simulink model "TEST_LIDAR"  (R2022b)
settings: Solver=FixedStepAuto  StartTime=0.0  StopTime=inf  FixedStep=1e-3  RelTol=1e-3  EnableMultiTasking=on
model workspace (MAT data in the model file):
  SL_ROS_VariableLengthArrays_MaxSizes : object (value not decoded)
values from neighbouring files (symbols this model uses):
  data = theClient.GetLastFrameOfData()    [FuncMotive.m]
undefined symbols (not defined in the file or in its folder): angular, carstamp, CIRCUIT, CLTF_DAMP, CLTF_FREQ, CLTF_GAIN, CONTROL, CONTROL_INI, DiscIntNeverNeededParam, INPUT, linear, MCP3201, MD25, MODEL, MODEL_INI, mpcstate, MPU60X0, MPU9250, MSG, NAV_MPC_CONTROL, OUTPUT, RCRX, SAMPLING_TIME, SYSID_INPUT, VL6180X
libraries: raspberrypiCommlib x160, simulink x89, raspberrypiNetworklib x22, ros2lib x14, dspsigattribs x14, embedlinuxBasiclib x12, ctrlSharedLib x2, mpclib x1, vrlib x1, sldrtlib x1
(part 14 of 19)

== matlab function TEST_LIDAR/HARDWARE/SENSORS/RCRX iBUS/BUS UPDATE ==
  data: CONTROL_IN input; CONTROL output Bus: CONTROL_Bus; CH_RAW input size=14
function CONTROL = RCRX_UPDATE(CONTROL_IN,CH_RAW)
%--------------------------------------------------------------
% COPY CONTROL BUS
CONTROL = CONTROL_IN;
%--------------------------------------------------------------
% SCALING PARAMETERS
% Open-loop RC scale {'COM MOTOR VOLT','DIFF MOTOR VOLT'}
OPL_RC_SCALE = CONTROL.PARAM.OPL_RC_SCALE;
% Velocity RC scale {'FORWARD VEL REF','YAW RATE REF'}
VEL_RC_SCALE = CONTROL.PARAM.VEL_RC_SCALE;
% Wall follower RC scale {'FORWARD VEL REF','WALL DIST REF'}
WFL_RC_SCALE = CONTROL.PARAM.WFL_RC_SCALE;
% Navigation RC scale {'INC POS X REF','INC POS Y REF'}
NAV_RC_SCALE = CONTROL.PARAM.NAV_RC_SCALE;
%--------------------------------------------------------------
% CHANNEL CALIBRATION
CALIB_PARAM = CONTROL.PARAM.RC_CALIB_PARAM;
CH_TRIM = CONTROL.PARAM.RC_CH_TRIM;
NUM_CH = length(CH_RAW);
CH_PU = zeros(NUM_CH,1);
CH_RAW = double(CH_RAW);
for nn = 1:NUM_CH
    CH_PU(nn) = (CALIB_PARAM(nn,1)*CH_RAW(nn) + CALIB_PARAM(nn,2)).*double(CH_RAW(nn)<CH_TRIM(nn)) + ...
                (CALIB_PARAM(nn,3)*CH_RAW(nn) + CALIB_PARAM(nn,4)).*double(CH_RAW(nn)>=CH_TRIM(nn));
end        
% Channel definition : {'COM MOTOR VOLT','DIFF MOTOR VOLT'}
%                      {'FORWARD VEL REF','YAW RATE REF'}
%                      {'FORWARD VEL REF','YAW ANGLE REF'}
%                      {'FORWARD VEL REF','WALL DIST REF'}
%                      {'INC POS X REF','INC POS Y REF'}
CH_DEF = CONTROL.PARAM.RC_CH_DEF;
% Throttle channel between 0 and 1 
% CH_PU(CH_DEF(4)) = (CH_PU(CH_DEF(4))+1)/2; 
%--------------------------------------------------------------
% TARGET DEFINITION
switch CONTROL.STATE.CONTROL_MODE 
    case 0 % OPEN LOOP
        % {'COMMON MOTOR VOLT','DIFFERENTIAL MOTOR VOLT'}
        if CONTROL.STATE.MV_TARGET_SOURCE(1)==2 % JOYSTICK
            CONTROL.TARGET.MOTOR_VOLT_CD_REF_RC(1) = CH_PU(CH_DEF(1))*OPL_RC_SCALE(1);
        end
        if CONTROL.STATE.MV_TARGET_SOURCE(2)==2 % JOYSTICK
            CONTROL.TARGET.MOTOR_VOLT_CD_REF_RC(2) = CH_PU(CH_DEF(2))*OPL_RC_SCALE(2);
        end
        if CONTROL.STATE.MV_TARGET_SOURCE(1)==3 % SWITCH
            CONTROL.TARGET.MOTOR_VOLT_CD_REF_RC(1) = CONTROL.PARAM.OPL_RC_SWITCH(1,round(2+CH_PU(5)));
        end
        if CONTROL.STATE.MV_TARGET_SOURCE(2)==3 % SWITCH
            CONTROL.TARGET.MOTOR_VOLT_CD_REF_RC(2) = CONTROL.PARAM.OPL_RC_SWITCH(2,round(2+CH_PU(6)));
        end       
    case 1 % FORWARD VELOCITY AND YAW ANGLE
        % {'FORWARD VEL REF','YAW ANGLE REF'}
        if CONTROL.STATE.FV_TARGET_SOURCE==2 % JOYSTICK
            CONTROL.TARGET.FORWARD_VEL_REF_RC = CH_PU(CH_DEF(1))*VEL_RC_SCALE(1);
        end
        if CONTROL.STATE.YA_TARGET_SOURCE==2 % JOYSTICK
            CONTROL.TARGET.YAW_ANG_REF_RC = CH_PU(CH_DEF(2))*VEL_RC_SCALE(2);
        end
        if CONTROL.STATE.FV_TARGET_SOURCE==3 % SWITCH
            CONTROL.TARGET.FORWARD_VEL_REF_RC = CONTROL.PARAM.VEL_RC_SWITCH(1,round(2+CH_PU(5)));
        end
        if CONTROL.STATE.YA_TARGET_SOURCE==3 % SWITCH
            CONTROL.TARGET.YAW_ANG_REF_RC = CONTROL.PARAM.VEL_RC_SWITCH(2,round(2+CH_PU(6)));
        end
    case 2 % FORWARD VELOCITY AND YAW RATE
        % {'FORWARD VEL REF','YAW RATE REF'}
        if CONTROL.STATE.FV_TARGET_SOURCE==2 % JOYSTICK
            CONTROL.TARGET.FORWARD_VEL_REF_RC = CH_PU(CH_DEF(1))*VEL_RC_SCALE(1);
        end
        if CONTROL.STATE.YR_TARGET_SOURCE==2 % JOYSTICK
            CONTROL.TARGET.YAW_RATE_REF_RC = CH_PU(CH_DEF(2))*VEL_RC_SCALE(2);
        end
        if CONTROL.STATE.FV_TARGET_SOURCE==3 % SWITCH
            CONTROL.TARGET.FORWARD_VEL_REF_RC = CONTROL.PARAM.VEL_RC_SWITCH(1,round(2+CH_PU(5)));
        end
        if CONTROL.STATE.YR_TARGET_SOURCE==3 % SWITCH
            CONTROL.TARGET.YAW_RATE_REF_RC = CONTROL.PARAM.VEL_RC_SWITCH(2,round(2+CH_PU(6)));
        end
    case 3 % NAVIGATION
        % {'INC POS X REF','INC POS Y REF'}
        if CONTROL.STATE.NAV_TARGET_SOURCE==2 % JOYSTICK
            CONTROL.TARGET.NAV_REF_RC(1) = CONTROL.INPUT.NAV_MO(1) + CH_PU(CH_DEF(1))*NAV_RC_SCALE;
            CONTROL.TARGET.NAV_REF_RC(2) = CONTROL.INPUT.NAV_MO(2) + CH_PU(CH_DEF(1))*NAV_RC_SCALE;
        end
        if CONTROL.STATE.NAV_TARGET_SOURCE==3 % SWITCH
            % CONTROL.TARGET.NAV_REF_RC(1) = CONTROL.INPUT.NAV_MO(1) + CONTROL.PARAM.NAV_RC_SWITCH(1,round(2+CH_PU(5)));
            % CONTROL.TARGET.NAV_REF_RC(2) = CONTROL.INPUT.NAV_MO(2) + CONTROL.PARAM.NAV_RC_SWITCH(2,round(2+CH_PU(6)));
            CONTROL.TARGET.NAV_REF_RC(1) = CONTROL.PARAM.NAV_RC_SWITCH(1,round(2+CH_PU(5)));
            CONTROL.TARGET.NAV_REF_RC(2) = CONTROL.PARAM.NAV_RC_SWITCH(2,round(2+CH_PU(6)));
        end
    case {4,5} % WALL FOLLOWER
        % {'FORWARD VEL REF','WALL DIST REF'}
        if CONTROL.STATE.FV_TARGET_SOURCE==2 % JOYSTICK
            CONTROL.TARGET.FORWARD_VEL_REF_RC = CH_PU(CH_DEF(1))*WFL_RC_SCALE(1);
        end
        % {'FORWARD VEL REF','WALL DIST REF'}
        if CONTROL.STATE.WD_TARGET_SOURCE==2 % JOYSTICK
            CONTROL.TARGET.WALL_DIST_REF_RC = 0.1 + CH_PU(CH_DEF(2))*WFL_RC_SCALE(2);
        end
        if CONTROL.STATE.FV_TARGET_SOURCE==3 % SWITCH
            CONTROL.TARGET.FORWARD_VEL_REF_RC = CONTROL.PARAM.WFL_RC_SWITCH(1,round(2+CH_PU(5)));
        end
        if CONTROL.STATE.WD_TARGET_SOURCE==3 % SWITCH
            CONTROL.TARGET.WALL_DIST_REF_RC = CONTROL.PARAM.WFL_RC_SWITCH(2,round(2+CH_PU(6)));
        end
    otherwise % FORWARD VELOCITY AND YAW RATE
        % {'FORWARD VEL REF','YAW RATE REF'}
        if CONTROL.STATE.FV_TARGET_SOURCE==2 % JOYSTICK
            CONTROL.TARGET.FORWARD_VEL_REF_RC = CH_PU(CH_DEF(1))*VEL_RC_SCALE(1);
        end
        if CONTROL.STATE.YR_TARGET_SOURCE==2 % JOYSTICK
            CONTROL.TARGET.YAW_RATE_REF_RC = CH_PU(CH_DEF(2))*VEL_RC_SCALE(1);
        end
        if CONTROL.STATE.FV_TARGET_SOURCE==3 % SWITCH
            CONTROL.TARGET.FORWARD_VEL_REF_RC = CONTROL.PARAM.VEL_RC_SWITCH(1,round(2+CH_PU(5)));
        end
        if CONTROL.STATE.YR_TARGET_SOURCE==3 % SWITCH
            CONTROL.TARGET.YAW_RATE_REF_RC = CONTROL.PARAM.VEL_RC_SWITCH(2,round(2+CH_PU(6)));
        end
end
if abs(CONTROL.TARGET.MOTOR_VOLT_CD_REF_RC(1))<0.25
    CONTROL.TARGET.MOTOR_VOLT_CD_REF_RC(1) = 0;
end
if abs(CONTROL.TARGET.MOTOR_VOLT_CD_REF_RC(2))<0.25
    CONTROL.TARGET.MOTOR_VOLT_CD_REF_RC(2) = 0;
end
if abs(CONTROL.TARGET.FORWARD_VEL_REF_RC)<0.05
    CONTROL.TARGET.FORWARD_VEL_REF_RC = 0;
end
if abs(CONTROL.TARGET.YAW_RATE_REF_RC)<0.025
    CONTROL.TARGET.YAW_RATE_REF_RC = 0;
end
%--------------------------------------------------------------
% CONTROL BUS UPDATE
% RC CHANNELS (pu): channel range [-1 1] / Throtle range (channel 4) [0 1] 
CONTROL.TARGET.RC_CH_PU = CH_PU(:);
CONTROL.TARGET.RC_CH_RAW = CH_RAW(:);

== matlab function TEST_LIDAR/HARDWARE/SENSORS/RCRX iBUS/MATLAB Function ==
  data: iBUS_DATA input; CH_RAW output size=14
function CH_RAW = iBUS_DECODER(iBUS_DATA)
%--------------------------------------------------------------
persistent initialize CH_RAW_PREV
if isempty(initialize)
    initialize = 1;
    CH_RAW_PREV = uint16(1500*ones(14,1));
end
%--------------------------------------------------------------
% iBUS protocol: 14 channels uint16 in the range [1000 - 2000]
%--------------------------------------------------------------
% HEADER DETECTION
header = uint8([32 64]);
AUX1 = (iBUS_DATA == header(1));
AUX2 = (iBUS_DATA == header(2));
AUX3 = AUX1(1:end-1) & AUX2(2:end);
[max_value,index] = max(AUX3);
%--------------------------------------------------------------
% CHANNEL DETECTION
if max_value && ((index(1)+2+2*14-1)<=length(iBUS_DATA))
    CH_DATA = iBUS_DATA((index(1)+2):(index(1)+2+2*14-1));
    CH_LSB = uint16(CH_DATA(1:2:length(CH_DATA)));
    CH_MSB = uint16(CH_DATA(2:2:length(CH_DATA)));
    CH_RAW_AUX = uint16(CH_MSB*2^8 + CH_LSB);
    CH_RAW_PREV = CH_RAW_AUX;
else
    CH_RAW_AUX = CH_RAW_PREV;
end

CH_RAW = CH_RAW_AUX(1:14);

return

== matlab function TEST_LIDAR/GAZEBO SIMULATION/COMMUNICATIONS/BT_RX/MCS RX ==
  data: CONTROL_IN input; BUFFER_RX_LAST input; CONTROL output Bus: CONTROL_Bus; STATUS input
function CONTROL  = MCS_DECODER(CONTROL_IN,BUFFER_RX_LAST,STATUS)
                 
persistent BUFFER_RX PAYLOAD
if isempty(BUFFER_RX)
    BUFFER_RX = zeros(50,3,'uint8');
    PAYLOAD = zeros(26,1,'uint8');
end

% Initialization
MESSAGE_LEN = length(PAYLOAD);
CONTROL = CONTROL_IN;
[BUFFER_ROW,BUFFER_COL] = size(BUFFER_RX);
% Update buffer
BUFFER_RX_VEC = [BUFFER_RX(:) ; BUFFER_RX_LAST];
BUFFER_LEN = length(BUFFER_RX_VEC);
% Identify sequences [13 10 254]
IDX_AUX = find(BUFFER_RX_VEC(1:end-2)==uint8(13) & BUFFER_RX_VEC(2:end-1)==uint8(10) & BUFFER_RX_VEC(3:end)==uint8(254));
if isempty(IDX_AUX) 
    % There is not any message
    flag_msg = false;
    BUFFER_RX = zeros(size(BUFFER_RX),'uint8');
    return
elseif IDX_AUX(1)+MESSAGE_LEN+2>BUFFER_LEN 
    % There is 1 incomplete message 
    flag_msg = false;
    BUFFER_RX = [BUFFER_RX(:,2:end)  BUFFER_RX_LAST];
    return
else
    % There is 1 complete message at least  
    flag_msg = true;
    IDX_START = zeros(size(IDX_AUX));
    IDX_END = zeros(size(IDX_AUX));
    IDX_AUX = [IDX_AUX ; BUFFER_LEN];
    IDX_START(1) = IDX_AUX(1) + 3;
    IDX_END(1) = IDX_START(1) + MESSAGE_LEN - 1;    
    COUNT = 1;
    % The rest of sequences [13 10 254] are verified
    for nn = 2:length(IDX_AUX)-1
        if (IDX_END(COUNT) < IDX_AUX(nn)) && (IDX_AUX(nn)+3<BUFFER_LEN)
            if IDX_AUX(nn) + MESSAGE_LEN + 1 <= BUFFER_LEN
                COUNT = COUNT +1;
                IDX_START(COUNT) = IDX_AUX(nn) + 3;
                IDX_END(COUNT) = IDX_START(COUNT) + MESSAGE_LEN - 1;       
            end
        end
    end
end
IDX_START = IDX_START(1:COUNT);
IDX_END = IDX_END(1:COUNT);
% Message identification
NUM_MESSAGES = COUNT;
MESSAGE = cell(NUM_MESSAGES,1);
for COUNT = 1:NUM_MESSAGES
    % Message building
    MESSAGE{COUNT} = BUFFER_RX_VEC(IDX_START(COUNT):IDX_END(COUNT));
end
% Update BUFFER_RX
BUFFER_RX_VEC = [zeros(IDX_END(end)-BUFFER_ROW-1,1,'uint8') ; BUFFER_RX_VEC(IDX_END(end):end)];
for nn = 1:BUFFER_COL
    BUFFER_RX(:,nn) = BUFFER_RX_VEC((nn-1)*BUFFER_ROW+1:BUFFER_ROW*nn);
end

%%%%%%%%%%%%%%%%%%%%%%%%%%%%%%%%%%%%%%%%%%%%%%%%%%%%%%%%%%%%%%%%%%%%%%%%%%%
% MCS MESSAGES
%%%%%%%%%%%%%%%%%%%%%%%%%%%%%%%%%%%%%%%%%%%%%%%%%%%%%%%%%%%%%%%%%%%%%%%%%%%
if flag_msg && STATUS==0
    PAYLOAD(1:MESSAGE_LEN) = uint8(MESSAGE{end});
end
% CRC    
CRC_VALUE=uint16(65535);
for nn=1:MESSAGE_LEN-2
    TMP=bitxor(uint16(PAYLOAD(nn)),bitand(CRC_VALUE,uint16(255)));
    TMP4=bitand(bitshift(TMP,4),uint16(255));
    TMP=bitxor(TMP,TMP4);
    TMP8=bitshift(TMP,8);
    TMP3=bitshift(TMP,3);
    TMP_4=bitshift(TMP,-4);
    CRC_VALUE=bitxor(bitshift(CRC_VALUE,-8),bitxor(TMP8,bitxor(TMP3,TMP_4)));
    CRC_VALUE=bitand(CRC_VALUE,uint16(65535));
end
CRC1=uint8(bitand(CRC_VALUE,uint16(255)));
CRC2=uint8(bitand(bitshift(CRC_VALUE,-8),uint16(255)));

% CRC checking
if (CRC1 == PAYLOAD(MESSAGE_LEN-1))  && (CRC2 == PAYLOAD(MESSAGE_LEN))
    % WRITE IN THE CONTROL BUS
    CONTROL.INPUT.MCS_EARTH_POS(1) = double(typecast(PAYLOAD(1:4),'single'));
    CONTROL.INPUT.MCS_EARTH_POS(2) = double(typecast(PAYLOAD(5:8),'single'));
    CONTROL.INPUT.MCS_EARTH_POS(3) = double(typecast(PAYLOAD(9:12),'single'));
    CONTROL.INPUT.MCS_EULER_ANG(1) = double(typecast(PAYLOAD(13:16),'single'));
    CONTROL.INPUT.MCS_EULER_ANG(2) = double(typecast(PAYLOAD(17:20),'single'));
    CONTROL.INPUT.MCS_EULER_ANG(3) = double(typecast(PAYLOAD(21:24),'single'));

    % UNWRAPPING
    aux1 = CONTROL.INPUT.MCS_EULER_ANG(3);
    aux2 = CONTROL.TARGET.YAW_ANG_REF;
    INC_ANG = zeros(41,1);
    INC_ANG(1) = aux1-aux2;
    for ii = 1:20
        INC_ANG(2*ii)   = aux1-aux2-2*ii*pi;
        INC_ANG(2*ii+1) = aux1-aux2+2*ii*pi;
    end
    [~,ind] = min(abs(INC_ANG));
    NAV_YAW_ANG = aux2 + INC_ANG(ind);
    CONTROL.INPUT.MCS_EULER_ANG(3) = NAV_YAW_ANG;

    % POSITION CORRECTION
    % rv = rm + rc*exp(Shi*j)
    % xv = xm + xc*cos(Shi);
    % yv = ym + yc*sin(Shi);
    CONTROL.INPUT.MCS_EARTH_POS(1) = CONTROL.INPUT.MCS_EARTH_POS(1) - CONTROL.PARAM.NAV_CENTER_POS(1)*cos(CONTROL.INPUT.MCS_EULER_ANG(3));
    CONTROL.INPUT.MCS_EARTH_POS(2) = CONTROL.INPUT.MCS_EARTH_POS(2) - CONTROL.PARAM.NAV_CENTER_POS(2)*sin(CONTROL.INPUT.MCS_EULER_ANG(3));

    % INITIAL POSITION COMPENSATION
    if CONTROL.STATE.CURRENT_STATUS_SYS>1
        CONTROL.INPUT.MCS_EARTH_POS = CONTROL.INPUT.MCS_EARTH_POS - CONTROL.PARAM.MCS_EARTH_POS_OFFS;
        CONTROL.INPUT.MCS_EULER_ANG = CONTROL.INPUT.MCS_EULER_ANG - CONTROL.PARAM.MCS_EULER_ANG_OFFS;
    end
    
end
%%%%%%%%%%%%%%%%%%%%%%%%%%%%%%%%%%%%%%%%%%%%%%%%%%%%%%%%%%%%%%%%%%%%%%%%%%%


return

== matlab function TEST_LIDAR/CONTROL/LOCAL TARGETS/FORWARD VELOCITY TARGET/ PULSE GENERATION ==
  data: CONTROL input Bus: CONTROL_Bus; FORWARD_VEL_REF output
function FORWARD_VEL_REF = PULSE_GEN(CONTROL)
    
persistent TIMER initialize
if isempty(initialize)
    TIMER = 0;
    initialize = 1;
end

% SAMPLING TIME
SAMPLING_TIME = CONTROL.PARAM.SAMPLING_TIME; % s

%% OPERATION MODE
% / 0. BOOTING   / 1. SENSOR CALIBRATION / 2. READY
% / 3. OPEN LOOP / 4. ATTITUDE / 5. VELOCITY / 6. NAVIGATION / 
% / 7. WALL FOLLOWER / 8. WALL-FOLLOWER COMPETITION / 
% / 9. NAVIGATION COMPETITION / 10. STOP
CURRENT_STATUS = CONTROL.STATE.CURRENT_STATUS_SYS;
PREVIOUS_STATUS = CONTROL.STATE.PREVIOUS_STATUS;

if (CURRENT_STATUS == 5) && (PREVIOUS_STATUS == 5)   
    if TIMER > 7.5
        FORWARD_VEL_REF = 0;
    elseif TIMER < 5
        FORWARD_VEL_REF = 0;
        TIMER = TIMER + SAMPLING_TIME;
    else % 5 <= TIMER <= 7.5
        FORWARD_VEL_REF = 0.25;
        TIMER = TIMER + SAMPLING_TIME;
    end
else
    FORWARD_VEL_REF = 0;
    TIMER = 0;
end

== matlab function TEST_LIDAR/CONTROL/LOCAL TARGETS/YAW RATE TARGET/ PULSE GENERATION  ==
  data: CONTROL input Bus: CONTROL_Bus; YAW_RATE_REF output
function YAW_RATE_REF = PULSE_GEN(CONTROL)
    
persistent TIMER initialize
if isempty(initialize)
    TIMER = 0;
    initialize = 1;
end

% SAMPLING TIME
SAMPLING_TIME = CONTROL.PARAM.SAMPLING_TIME; % s

%% OPERATION MODE
% / 0. BOOTING   / 1. SENSOR CALIBRATION / 2. READY
% / 3. OPEN LOOP / 4. ATTITUDE / 5. VELOCITY / 6. NAVIGATION / 
% / 7. WALL FOLLOWER / 8. WALL-FOLLOWER COMPETITION / 
% / 9. NAVIGATION COMPETITION / 10. STOP
CURRENT_STATUS = CONTROL.STATE.CURRENT_STATUS_SYS;
PREVIOUS_STATUS = CONTROL.STATE.PREVIOUS_STATUS;

if (CURRENT_STATUS == 5) && (PREVIOUS_STATUS == 5)   
    if TIMER > 7.5
        YAW_RATE_REF = 0;
    elseif TIMER < 5
        YAW_RATE_REF = 0;
        TIMER = TIMER + SAMPLING_TIME;
    else % 5 <= TIMER <= 7.5
        YAW_RATE_REF = 30*pi/180;
        TIMER = TIMER + SAMPLING_TIME;
    end
else
    YAW_RATE_REF = 0;
    TIMER = 0;
end

== matlab function TEST_LIDAR/SIMULATION/CIRCUIT SIMULATION ==
  data: MODEL_IN input; MODEL output Bus: MODEL_Bus
function MODEL = CIRCUIT_SIM(MODEL_IN)
% function [d,theta_circ,d1,d2,rampa,estado] = CIRCUIT_SIM(xi,yi,theta,param,est_ant)

% PARAMETERS
MODEL.CIRCUIT.PERIMETER_POINTS = 1000;
MODEL.CIRCUIT.STRAIGHT_SIDE_LENGTH = 2;
MODEL.CIRCUIT.RAMP_LENGTH = 1.5;
MODEL.CIRCUIT.CURVE_RADIUS = 0.5;
MODEL.CIRCUIT.RAMP = 0;
MODEL.CIRCUIT.STATUS = 0;

L=param(1); % Longitud tramo recto
Lr=param(2); % Longitud rampa
R=param(3);  % Radio de la curva
d_sens=param(4); % Distancia entre sensores

% Sensor delantero
xid=xi+d_sens/2*cos(theta);
yid=yi+d_sens/2*sin(theta);
% Sensor trasero
xit=xi-d_sens/2*cos(theta);
yit=yi-d_sens/2*sin(theta);
% Ecuacion de la recta normal
% y-yi = tan(theta-pi/2)*(x-xi)

%% Distancia del sensor delantero
% Corte con el tramo recto de la pared del circuito
% x=xi+(sign(yi)*R-yi)/tan(theta-pi/2)
x_1=[xid+(R-yid)/tan(theta-pi/2); xid+(-R-yid)/tan(theta-pi/2)];
y_1=[R; -R];
V1=(x_1-xid)+1j*(y_1-yid);
V2=d_sens/2*cos(theta)+1j*d_sens/2*sin(theta);
ang_1=angle(V2./V1)*180/pi;
[~,ind]=min(abs(ang_1-90));
x_1=x_1(ind);
y_1=y_1(ind);
% Corte con la curva del circuito
% (yi+tan(theta-pi/2)*(x-xi))^2 = R^2-(x-sign(xi)*L/2)^2
% yi^2+tan(theta-pi/2)^2*(x^2+xi^2-2*xi*x)+2*tan(theta-pi/2)*(x-xi)*yi = R^2-x^2-L^2/4+2*sign(xi)*L/2*x
% x = roots([tan(theta-pi/2)^2+1  -2*(xi*tan(theta-pi/2)^2+sign(xi)*L/2-tan(theta-pi/2)*yi)   yi^2+tan(theta-pi/2)^2*xi^2-R^2+L^2/4-2*tan(theta-pi/2)*xi*yi])
if abs(x_1)<=L/2
    xcd=x_1;
    ycd=y_1;
else
    x_2 = roots([tan(theta-pi/2)^2+1 ...
        -2*(xid*tan(theta-pi/2)^2+sign(xid)*L/2-tan(theta-pi/2)*yid) ...
        yid^2+tan(theta-pi/2)^2*xid^2-R^2+L^2/4-2*tan(theta-pi/2)*xid*yid]);
        [~,ind]=min(abs(x_2-xid));
    xcd=x_2(ind);
    aux=sqrt(abs(R^2-(xcd-sign(xid)*L/2)^2));
    y_2=[aux ; -aux];
    V1=[(xcd-xid)+1j*(y_2(1)-yid) ; (xcd-xid)+1j*(y_2(2)-yid)];
    V2=[d_sens/2*cos(theta)+1j*d_sens/2*sin(theta); d_sens/2*cos(theta)+1j*d_sens/2*sin(theta)];
    ang_2=angle(V2./V1)*180/pi;
    [~,ind]=min(abs(ang_2-90));
    ycd=y_2(ind);
end
d1=norm([xcd-xid ; ycd-yid]);

%% Distancia del sensor trasero
% Corte con el tramo recto de la pared del circuito
% x=xi+(sign(yi)*R-yi)/tan(theta-pi/2)
x_1=[xit+(R-yit)/tan(theta-pi/2); xit+(-R-yit)/tan(theta-pi/2)];
y_1=[R; -R];
V1=(x_1-xit)+1j*(y_1-yit);
V2=d_sens/2*cos(theta)+1j*d_sens/2*sin(theta);
ang_1=angle(V2./V1)*180/pi;
[~,ind]=min(abs(ang_1-90));
x_1=x_1(ind);
y_1=y_1(ind);
% Corte con la curva del circuito
% (yi+tan(theta-pi/2)*(x-xi))^2 = R^2-(x-sign(xi)*L/2)^2
% yi^2+tan(theta-pi/2)^2*(x^2+xi^2-2*xi*x)+2*tan(theta-pi/2)*(x-xi)*yi = R^2-x^2-L^2/4+2*sign(xi)*L/2*x
% x = roots([tan(theta-pi/2)^2+1  -2*(xi*tan(theta-pi/2)^2+sign(xi)*L/2-tan(theta-pi/2)*yi)   yi^2+tan(theta-pi/2)^2*xi^2-R^2+L^2/4-2*tan(theta-pi/2)*xi*yi])
if abs(x_1)<=L/2
    xct=x_1;
    yct=y_1;
else
    x_2 = roots([tan(theta-pi/2)^2+1 ...
        -2*(xit*tan(theta-pi/2)^2+sign(xit)*L/2-tan(theta-pi/2)*yit) ...
        yit^2+tan(theta-pi/2)^2*xit^2-R^2+L^2/4-2*tan(theta-pi/2)*xit*yit]);
        [~,ind]=min(abs(x_2-xit));
    xct=x_2(ind);
    aux=sqrt(abs(R^2-(xct-sign(xit)*L/2)^2));
    y_2=[aux ; -aux];
    V1=[(xct-xit)+1j*(y_2(1)-yit) ; (xct-xit)+1j*(y_2(2)-yit)];
    V2=[d_sens/2*cos(theta)+1j*d_sens/2*sin(theta); d_sens/2*cos(theta)+1j*d_sens/2*sin(theta)];
    ang_2=angle(V2./V1)*180/pi;
    [~,ind]=min(abs(ang_2-90));
    yct=y_2(ind);
end
d2=norm([xct-xit ; yct-yit]);

%% Angulo con respecto al circuito
theta_circ=atan2(d1-d2,d_sens);

%% Distancia en m
d=(d1+d2)/2/cosd(theta_circ);
d1=d1;
d2=d2;

% Existencia de rampa
rampa=0;
if abs(xi)<=Lr/2 
   % El coche está en la rampa
   if yi<0
       % Rampa ascendente
       rampa=1;
   else
       % Rampa descendente
       rampa=-1;
   end
end
% Determinacion del estado
if abs(xi)<=L/2 
   % El coche está en el tramo recto
   if yi<0
       % Subida
       estado=est_ant+(rem(est_ant,4)==1);
   else
       % Bajada
       estado=est_ant+(rem(est_ant,4)==3);
   end
elseif xi>L/2
    % El coche está en la curva superior
       estado=est_ant+(rem(est_ant,4)==2);
else
    % El coche está en la curva inferior
    estado=est_ant+(rem(est_ant,4)==0);
end

== matlab function TEST_LIDAR/HARDWARE/COMMUNICATIONS/BT_RX/MCS RX ==
  data: CONTROL_IN input; BUFFER_RX_LAST input; CONTROL output Bus: CONTROL_Bus; STATUS input
function CONTROL  = MCS_DECODER(CONTROL_IN,BUFFER_RX_LAST,STATUS)
                 
persistent BUFFER_RX PAYLOAD
if isempty(BUFFER_RX)
    BUFFER_RX = zeros(50,3,'uint8');
    PAYLOAD = zeros(26,1,'uint8');
end

% Initialization
MESSAGE_LEN = length(PAYLOAD);
CONTROL = CONTROL_IN;
[BUFFER_ROW,BUFFER_COL] = size(BUFFER_RX);
% Update buffer
BUFFER_RX_VEC = [BUFFER_RX(:) ; BUFFER_RX_LAST];
BUFFER_LEN = length(BUFFER_RX_VEC);
% Identify sequences [13 10 254]
IDX_AUX = find(BUFFER_RX_VEC(1:end-2)==uint8(13) & BUFFER_RX_VEC(2:end-1)==uint8(10) & BUFFER_RX_VEC(3:end)==uint8(254));
if isempty(IDX_AUX) 
    % There is not any message
    flag_msg = false;
    BUFFER_RX = zeros(size(BUFFER_RX),'uint8');
    return
elseif IDX_AUX(1)+MESSAGE_LEN+2>BUFFER_LEN 
    % There is 1 incomplete message 
    flag_msg = false;
    BUFFER_RX = [BUFFER_RX(:,2:end)  BUFFER_RX_LAST];
    return
else
    % There is 1 complete message at least  
    flag_msg = true;
    IDX_START = zeros(size(IDX_AUX));
    IDX_END = zeros(size(IDX_AUX));
    IDX_AUX = [IDX_AUX ; BUFFER_LEN];
    IDX_START(1) = IDX_AUX(1) + 3;
    IDX_END(1) = IDX_START(1) + MESSAGE_LEN - 1;    
    COUNT = 1;
    % The rest of sequences [13 10 254] are verified
    for nn = 2:length(IDX_AUX)-1
        if (IDX_END(COUNT) < IDX_AUX(nn)) && (IDX_AUX(nn)+3<BUFFER_LEN)
            if IDX_AUX(nn) + MESSAGE_LEN + 1 <= BUFFER_LEN
                COUNT = COUNT +1;
                IDX_START(COUNT) = IDX_AUX(nn) + 3;
                IDX_END(COUNT) = IDX_START(COUNT) + MESSAGE_LEN - 1;       
            end
        end
    end
end
IDX_START = IDX_START(1:COUNT);
IDX_END = IDX_END(1:COUNT);
% Message identification
NUM_MESSAGES = COUNT;
MESSAGE = cell(NUM_MESSAGES,1);
for COUNT = 1:NUM_MESSAGES
    % Message building
    MESSAGE{COUNT} = BUFFER_RX_VEC(IDX_START(COUNT):IDX_END(COUNT));
end
% Update BUFFER_RX
BUFFER_RX_VEC = [zeros(IDX_END(end)-BUFFER_ROW-1,1,'uint8') ; BUFFER_RX_VEC(IDX_END(end):end)];
for nn = 1:BUFFER_COL
    BUFFER_RX(:,nn) = BUFFER_RX_VEC((nn-1)*BUFFER_ROW+1:BUFFER_ROW*nn);
end

%%%%%%%%%%%%%%%%%%%%%%%%%%%%%%%%%%%%%%%%%%%%%%%%%%%%%%%%%%%%%%%%%%%%%%%%%%%
% MCS MESSAGES
%%%%%%%%%%%%%%%%%%%%%%%%%%%%%%%%%%%%%%%%%%%%%%%%%%%%%%%%%%%%%%%%%%%%%%%%%%%
if flag_msg && STATUS==0
    PAYLOAD(1:MESSAGE_LEN) = uint8(MESSAGE{end});
end
% CRC    
CRC_VALUE=uint16(65535);
for nn=1:MESSAGE_LEN-2
    TMP=bitxor(uint16(PAYLOAD(nn)),bitand(CRC_VALUE,uint16(255)));
    TMP4=bitand(bitshift(TMP,4),uint16(255));
    TMP=bitxor(TMP,TMP4);
    TMP8=bitshift(TMP,8);
    TMP3=bitshift(TMP,3);
    TMP_4=bitshift(TMP,-4);
    CRC_VALUE=bitxor(bitshift(CRC_VALUE,-8),bitxor(TMP8,bitxor(TMP3,TMP_4)));
    CRC_VALUE=bitand(CRC_VALUE,uint16(65535));
end
CRC1=uint8(bitand(CRC_VALUE,uint16(255)));
CRC2=uint8(bitand(bitshift(CRC_VALUE,-8),uint16(255)));

% CRC checking
if (CRC1 == PAYLOAD(MESSAGE_LEN-1))  && (CRC2 == PAYLOAD(MESSAGE_LEN))
    % WRITE IN THE CONTROL BUS
    CONTROL.INPUT.MCS_EARTH_POS(1) = double(typecast(PAYLOAD(1:4),'single'));
    CONTROL.INPUT.MCS_EARTH_POS(2) = double(typecast(PAYLOAD(5:8),'single'));
    CONTROL.INPUT.MCS_EARTH_POS(3) = double(typecast(PAYLOAD(9:12),'single'));
    CONTROL.INPUT.MCS_EULER_ANG(1) = double(typecast(PAYLOAD(13:16),'single'));
    CONTROL.INPUT.MCS_EULER_ANG(2) = double(typecast(PAYLOAD(17:20),'single'));
    CONTROL.INPUT.MCS_EULER_ANG(3) = double(typecast(PAYLOAD(21:24),'single'));

    % UNWRAPPING
    aux1 = CONTROL.INPUT.MCS_EULER_ANG(3);
    aux2 = CONTROL.TARGET.YAW_ANG_REF;
    INC_ANG = zeros(41,1);
    INC_ANG(1) = aux1-aux2;
    for ii = 1:20
        INC_ANG(2*ii)   = aux1-aux2-2*ii*pi;
        INC_ANG(2*ii+1) = aux1-aux2+2*ii*pi;
    end
    [~,ind] = min(abs(INC_ANG));
    NAV_YAW_ANG = aux2 + INC_ANG(ind);
    CONTROL.INPUT.MCS_EULER_ANG(3) = NAV_YAW_ANG;

    % POSITION CORRECTION
    % rv = rm + rc*exp(Shi*j)
    % xv = xm + xc*cos(Shi);
    % yv = ym + yc*sin(Shi);
    CONTROL.INPUT.MCS_EARTH_POS(1) = CONTROL.INPUT.MCS_EARTH_POS(1) - CONTROL.PARAM.NAV_CENTER_POS(1)*cos(CONTROL.INPUT.MCS_EULER_ANG(3));
    CONTROL.INPUT.MCS_EARTH_POS(2) = CONTROL.INPUT.MCS_EARTH_POS(2) - CONTROL.PARAM.NAV_CENTER_POS(2)*sin(CONTROL.INPUT.MCS_EULER_ANG(3));

    % INITIAL POSITION COMPENSATION
    if CONTROL.STATE.CURRENT_STATUS_SYS>1
        CONTROL.INPUT.MCS_EARTH_POS = CONTROL.INPUT.MCS_EARTH_POS - CONTROL.PARAM.MCS_EARTH_POS_OFFS;
        CONTROL.INPUT.MCS_EULER_ANG = CONTROL.INPUT.MCS_EULER_ANG - CONTROL.PARAM.MCS_EULER_ANG_OFFS;
    end
    
end
%%%%%%%%%%%%%%%%%%%%%%%%%%%%%%%%%%%%%%%%%%%%%%%%%%%%%%%%%%%%%%%%%%%%%%%%%%%


return

== matlab function TEST_LIDAR/HARDWARE/ACTUATORS/MD25_I2C/READ BATTERY VOLTAGE/BATTERY VOLTAGE FILTER ==
  data: CONTROL_IN input; BATTERY_VOLT input; CONTROL output Bus: CONTROL_Bus; RATED_BATTERY_VOLT input; THR_NLFILT input; ALFA_FILT input
function CONTROL = BATTERY_VOLT_FILTER(CONTROL_IN,BATTERY_VOLT,RATED_BATTERY_VOLT,THR_NLFILT,ALFA_FILT)

%--------------------------------------------------------------
% COPY CONTROL BUS
%--------------------------------------------------------------
CONTROL = CONTROL_IN;

%--------------------------------------------------------------
% STATE
%--------------------------------------------------------------
persistent initialize BATTERY_VOLT_NLFILT BATTERY_VOLT_FILT
if isempty(initialize)
    BATTERY_VOLT_NLFILT = RATED_BATTERY_VOLT;
    BATTERY_VOLT_FILT = RATED_BATTERY_VOLT;
    initialize = 1;
end

%--------------------------------------------------------------
% NON-LINEAR FILTER
%--------------------------------------------------------------
if abs(BATTERY_VOLT - BATTERY_VOLT_NLFILT) < THR_NLFILT
    BATTERY_VOLT_NLFILT = BATTERY_VOLT;
end

%--------------------------------------------------------------
% FIRST-ORDER LINEAR FILTER
%--------------------------------------------------------------
BATTERY_VOLT_FILT = ALFA_FILT*BATTERY_VOLT_FILT + (1-ALFA_FILT)*BATTERY_VOLT_NLFILT;

%--------------------------------------------------------------
% CONTROL BUS UPDATE
%--------------------------------------------------------------
CONTROL.INPUT.BATTERY_VOLT = BATTERY_VOLT_FILT; % V   

return

== matlab function TEST_LIDAR/HARDWARE/ACTUATORS/MD25_I2C/READ MOTOR ENCODER/READ ENCODER ANGLE ==
  data: CONTROL_IN input; MOTOR_ENC_BYTES input uint8; CONTROL output CONTROL_Bus
function CONTROL = READ_ENCODER_ANGLE(CONTROL_IN,MOTOR_ENC_BYTES)

%--------------------------------------------------------------
% COPY CONTROL BUS
%--------------------------------------------------------------
CONTROL = CONTROL_IN;

%--------------------------------------------------------------
% PARAMETERS
%--------------------------------------------------------------
% Sampling time (s)
SAMPLING_TIME = CONTROL.PARAM.SAMPLING_TIME;
% Encoder filter frequency (Hz)
ENC_FILT_FREQ = CONTROL.PARAM.ENC_FILT_FREQ;
% Distance between wheeels (m)
WHEEL_DIST = CONTROL.PARAM.WHEEL_DISTANCE;
% Wheel radius (m)
WHEEL_RADIUS = CONTROL.PARAM.WHEEL_RADIUS;
% Wheel gear ratio
WHEEL_GEAR_RATIO = CONTROL.PARAM.WHEEL_GEAR_RATIO;
% Motor gear ratio
MOTOR_GEAR_RATIO = CONTROL.PARAM.MOTOR_GEAR_RATIO;
% Encoder resolution: number of pulses / revolution of main shaft
MOTOR_ENC_RES = CONTROL.PARAM.MOTOR_ENC_RES; 

%--------------------------------------------------------------
% ENCODER READOUT
%--------------------------------------------------------------
MOTOR_ENC_COUNT = zeros(2,1);
MOTOR_ENC_COUNT(1) = -double(typecast(MOTOR_ENC_BYTES([4 3 2 1],1),'int32'));
MOTOR_ENC_COUNT(2) = -double(typecast(MOTOR_ENC_BYTES([8 7 6 5],1),'int32'));

%--------------------------------------------------------------
% STATE
%--------------------------------------------------------------
persistent initialize INC_ENC_FILT ENC_COUNT_NLFILT YAW_ANGLE YAW_ANGLE_FILT...
           YAW_RATE YAW_RATE_FILT
if isempty(initialize)
    YAW_ANGLE = 0;
    YAW_RATE = 0;
    YAW_ANGLE_FILT = 0;
    YAW_RATE_FILT = 0;
    INC_ENC_FILT = zeros(2,1); 
    ENC_COUNT_NLFILT = MOTOR_ENC_COUNT;
    initialize = 1;
end

%--------------------------------------------------------------
% NON-LINEAR FILTER
%--------------------------------------------------------------
LAST_ENC_COUNT_NLFILT = ENC_COUNT_NLFILT;
MOTOR_ENC_COUNT_INC = MOTOR_ENC_COUNT - ENC_COUNT_NLFILT;
AUX = abs(MOTOR_ENC_COUNT)>0 & abs(MOTOR_ENC_COUNT_INC)<50;
if AUX(1)
    ENC_COUNT_NLFILT(1) = MOTOR_ENC_COUNT(1);
end
if AUX(2)
    ENC_COUNT_NLFILT(2) = MOTOR_ENC_COUNT(2);
end

%--------------------------------------------------------------
% LINEAR FILTER APPLIED TO INCREMENTAL ENCODER COUNT
%--------------------------------------------------------------
INC_ENC = ENC_COUNT_NLFILT - LAST_ENC_COUNT_NLFILT;
% LPF discrete-time pole
ALFA = exp(-SAMPLING_TIME*2*pi*ENC_FILT_FREQ);
INC_ENC_FILT = ALFA*INC_ENC_FILT + (1-ALFA)*INC_ENC;  

%--------------------------------------------------------------
% FORWARD VELOCITY
%--------------------------------------------------------------
FORWARD_VEL = mean(INC_ENC)/MOTOR_ENC_RES*2*pi/SAMPLING_TIME/MOTOR_GEAR_RATIO/WHEEL_GEAR_RATIO*WHEEL_RADIUS;
FORWARD_VEL_FILT = mean(INC_ENC_FILT)/MOTOR_ENC_RES*2*pi/SAMPLING_TIME/MOTOR_GEAR_RATIO/WHEEL_GEAR_RATIO*WHEEL_RADIUS;

%--------------------------------------------------------------
% YAW RATE
%--------------------------------------------------------------
YAW_RATE_PRV = YAW_RATE;
YAW_RATE_PRV_FILT = YAW_RATE_FILT;
YAW_RATE = (INC_ENC(1)-INC_ENC(2))/MOTOR_ENC_RES*2*pi/SAMPLING_TIME/MOTOR_GEAR_RATIO/WHEEL_GEAR_RATIO*WHEEL_RADIUS/WHEEL_DIST;
YAW_RATE_FILT = (INC_ENC_FILT(1)-INC_ENC_FILT(2))/MOTOR_ENC_RES*2*pi/SAMPLING_TIME/MOTOR_GEAR_RATIO/WHEEL_GEAR_RATIO*WHEEL_RADIUS/WHEEL_DIST;

%--------------------------------------------------------------
% YAW ANGLE
%--------------------------------------------------------------
YAW_ANGLE_PRV = YAW_ANGLE;
YAW_ANGLE_PRV_FILT = YAW_ANGLE_FILT;
YAW_ANGLE = YAW_ANGLE_PRV + SAMPLING_TIME/2*(YAW_RATE + YAW_RATE_PRV);
YAW_ANGLE_FILT = YAW_ANGLE_PRV_FILT + SAMPLING_TIME/2*(YAW_RATE_FILT + YAW_RATE_PRV_FILT);

%--------------------------------------------------------------
% MOTOR RATE
%--------------------------------------------------------------
MOTOR_RATE = INC_ENC/MOTOR_ENC_RES*2*pi/MOTOR_GEAR_RATIO/SAMPLING_TIME;
MOTOR_RATE_FILT = INC_ENC_FILT/MOTOR_ENC_RES*2*pi/MOTOR_GEAR_RATIO/SAMPLING_TIME;
MOTOR_RATE_CD = [sum(MOTOR_RATE) -diff(MOTOR_RATE)]/2;
MOTOR_RATE_CD_FILT = [sum(MOTOR_RATE_FILT) -diff(MOTOR_RATE_FILT)]/2;

%--------------------------------------------------------------
% UPDATE CONTROL BUS
%--------------------------------------------------------------
CONTROL.INPUT.ENC_FORWARD_VEL = FORWARD_VEL;
CONTROL.INPUT.ENC_FORWARD_VEL_FILT = FORWARD_VEL_FILT;
CONTROL.INPUT.ENC_YAW_RATE = YAW_RATE;
CONTROL.INPUT.ENC_YAW_RATE_FILT = YAW_RATE_FILT;
CONTROL.INPUT.ENC_YAW_ANG = YAW_ANGLE;
CONTROL.INPUT.ENC_YAW_ANG_FILT = YAW_ANGLE_FILT;
CONTROL.INPUT.ENC_MOTOR_RATE = MOTOR_RATE;
CONTROL.INPUT.ENC_MOTOR_RATE_FILT = MOTOR_RATE_FILT;
CONTROL.INPUT.ENC_MOTOR_RATE_CD = MOTOR_RATE_CD';
CONTROL.INPUT.ENC_MOTOR_RATE_CD_FILT = MOTOR_RATE_CD_FILT';
CONTROL.INPUT.ENC_MOTOR_ANG = ENC_COUNT_NLFILT/MOTOR_ENC_RES*2*pi/MOTOR_GEAR_RATIO;

== matlab function TEST_LIDAR/HARDWARE/ACTUATORS/MD25_I2C/WRITE PWM MOTOR /PWM CONVERSION ==
  data: PWM_BYTE output int8; CONTROL input Bus: CONTROL_Bus; PWM_MAX input; PWM_MIN input; MOTOR_PWM output
function [PWM_BYTE,MOTOR_PWM] = PWM_CONVERSION(CONTROL,PWM_MAX,PWM_MIN)

%--------------------------------------------------------------
% ENABLING MOTORS
%--------------------------------------------------------------
MOTOR_VOLT = CONTROL.OUTPUT.MOTOR_VOLT.*double(CONTROL.STATE.MOTOR_MODE);
% BATTERY_VOLT = CONTROL.INPUT.BATTERY_VOLT;

%--------------------------------------------------------------
% LIMITING MOTOR VOLTAGES
%--------------------------------------------------------------
% MOTOR_VOLT between -MOTOR_VOLT_MAX and MOTOR_VOLT_MAX
% MOTOR_VOLT_MAX = [BATTERY_VOLT BATTERY_VOLT]';
MOTOR_VOLT_MAX = CONTROL.PARAM.MOTOR_VOLT_MAX;
MOTOR_VOLT = MOTOR_VOLT.*(MOTOR_VOLT<MOTOR_VOLT_MAX & MOTOR_VOLT>-MOTOR_VOLT_MAX) + ...
           MOTOR_VOLT_MAX.*(MOTOR_VOLT>=MOTOR_VOLT_MAX) - MOTOR_VOLT_MAX.*(MOTOR_VOLT<=-MOTOR_VOLT_MAX);


%--------------------------------------------------------------
% PWM COMPUTATION
%--------------------------------------------------------------
PWM_AUX = zeros(2,1);
DEAD_ZONE = CONTROL.PARAM.MOTOR_DEAD_ZONE;
PWM_SLOPE = CONTROL.PARAM.MOTOR_PWM_SLOPE;
if MOTOR_VOLT(1)>=DEAD_ZONE(2)+2*PWM_SLOPE(2)
    PWM_AUX(1) = (MOTOR_VOLT(1)-DEAD_ZONE(2))/PWM_SLOPE(2);
elseif MOTOR_VOLT(1)<=DEAD_ZONE(1)-2*PWM_SLOPE(1)
    PWM_AUX(1) = (MOTOR_VOLT(1)-DEAD_ZONE(1))/PWM_SLOPE(1);
else
    PWM_AUX(1) = 0;
end
if MOTOR_VOLT(2)>=DEAD_ZONE(2)+2*PWM_SLOPE(2)
    PWM_AUX(2) = (MOTOR_VOLT(2)-DEAD_ZONE(2))/PWM_SLOPE(2);
elseif MOTOR_VOLT(2)<=DEAD_ZONE(1)-2*PWM_SLOPE(1)
    PWM_AUX(2) = (MOTOR_VOLT(2)-DEAD_ZONE(1))/PWM_SLOPE(1);
else
    PWM_AUX(2) = 0;
end

% PWM between PWM_MAX and PWM_MIN 
% PWM_AUX = (PWM_MAX-PWM_MIN)/2*(MOTOR_VOLT/BATTERY_VOLT - 1) + PWM_MAX;
PWM_AUX = PWM_AUX.*(PWM_AUX<PWM_MAX & PWM_AUX>PWM_MIN) + ...
          PWM_MAX*(PWM_AUX>=PWM_MAX) + PWM_MIN*(PWM_AUX<=PWM_MIN);      
PWM_BYTE = int8(-PWM_AUX);
% PWM in %
% MOTOR_PWM = MOTOR_VOLT/BATTERY_VOLT*100;
MOTOR_PWM = PWM_AUX/PWM_MAX*100;

== matlab function TEST_LIDAR/HARDWARE/COMMUNICATIONS/UART_MUX/BT MCS/MCS RX ==
  data: CONTROL_IN input; BUFFER_RX_LAST input; CONTROL output Bus: CONTROL_Bus
function CONTROL  = MCS_DECODER(CONTROL_IN,BUFFER_RX_LAST)
                 
persistent BUFFER_RX 
if isempty(BUFFER_RX)
    BUFFER_RX = zeros(50,3,'uint8');
end

% Initialization
CONTROL = CONTROL_IN;
MESSAGE_LEN = 24;
[BUFFER_ROW,BUFFER_COL] = size(BUFFER_RX);
% Update buffer
BUFFER_RX_VEC = [BUFFER_RX(:) ; BUFFER_RX_LAST];
BUFFER_LEN = length(BUFFER_RX_VEC);
% Identify sequences [0 254]
IDX_AUX = find(BUFFER_RX_VEC(1:end-1)==uint8(0) & BUFFER_RX_VEC(2:end)==uint8(254));
if isempty(IDX_AUX) 
    % There is not any message
    BUFFER_RX = zeros(size(BUFFER_RX),'uint8');
    return
elseif IDX_AUX(1)+MESSAGE_LEN+1>BUFFER_LEN 
    % There is 1 incomplete message 
    BUFFER_RX = [BUFFER_RX(:,2:end)  BUFFER_RX_LAST];
    return
else
    % There is 1 complete message at least    
    IDX_START = zeros(size(IDX_AUX));
    IDX_END = zeros(size(IDX_AUX));
    IDX_AUX = [IDX_AUX ; BUFFER_LEN];
    IDX_START(1) = IDX_AUX(1) + 2;
    IDX_END(1) = IDX_START(1) + MESSAGE_LEN - 1;    
    COUNT = 1;
    % The rest of sequences [0 254] are verified
    for nn = 2:length(IDX_AUX)-1
        if (IDX_END(COUNT) < IDX_AUX(nn)) && (IDX_AUX(nn)+2<BUFFER_LEN)
            if IDX_AUX(nn) + MESSAGE_LEN + 1 <= BUFFER_LEN
                COUNT = COUNT +1;
                IDX_START(COUNT) = IDX_AUX(nn) + 2;
                IDX_END(COUNT) = IDX_START(COUNT) + MESSAGE_LEN - 1;       
            end
        end
    end
end
IDX_START = IDX_START(1:COUNT);
IDX_END = IDX_END(1:COUNT);
% Message identification
NUM_MESSAGES = COUNT;
MESSAGE = cell(NUM_MESSAGES,1);
for COUNT = 1:NUM_MESSAGES
    % Message building
    MESSAGE{COUNT} = BUFFER_RX_VEC(IDX_START(COUNT):IDX_END(COUNT));
end
% Update BUFFER_RX
BUFFER_RX_VEC = [zeros(IDX_END(end)-BUFFER_ROW-1,1,'uint8') ; BUFFER_RX_VEC(IDX_END(end):end)];
for nn = 1:BUFFER_COL
    BUFFER_RX(:,nn) = BUFFER_RX_VEC((nn-1)*BUFFER_ROW+1:BUFFER_ROW*nn);
end

%%%%%%%%%%%%%%%%%%%%%%%%%%%%%%%%%%%%%%%%%%%%%%%%%%%%%%%%%%%%%%%%%%%%%%%%%%%
% MCS MESSAGES
%%%%%%%%%%%%%%%%%%%%%%%%%%%%%%%%%%%%%%%%%%%%%%%%%%%%%%%%%%%%%%%%%%%%%%%%%%%
PAYLOAD = uint8(MESSAGE{end});

% Escribir en el bus de control
CONTROL.INPUT.MCS_POS_XY(1) = typecast(PAYLOAD(1:8),'double');
CONTROL.INPUT.MCS_POS_XY(2) = typecast(PAYLOAD(9:16),'double');
MCS_YAW_ANG = typecast(PAYLOAD(17:24),'double');
% UNWRAPPING
aux1 = MCS_YAW_ANG;
aux2 = CONTROL.TARGET.YAW_ANG_REF;
INC_YAW_ANG = [aux1-aux2
               aux1-aux2-2*pi
               aux1-aux2+2*pi];
[~,ind] = min(abs(INC_YAW_ANG));
MCS_YAW_ANG = aux2 + INC_YAW_ANG(ind);

CONTROL.INPUT.MCS_YAW_ANG = MCS_YAW_ANG;
%%%%%%%%%%%%%%%%%%%%%%%%%%%%%%%%%%%%%%%%%%%%%%%%%%%%%%%%%%%%%%%%%%%%%%%%%%%


return

== matlab function TEST_LIDAR/HARDWARE/COMMUNICATIONS/UART_MUX/RCRX iBUS/BUS UPDATE ==
  data: CONTROL_IN input; CONTROL output Bus: CONTROL_Bus; CH_RAW input size=14; RCRX input
function CONTROL = RCRX_UPDATE(CONTROL_IN,CH_RAW,RCRX)
%--------------------------------------------------------------
% COPY CONTROL BUS
CONTROL = CONTROL_IN;
%--------------------------------------------------------------
% CHANNEL PARAMETERS
CH_MIN = RCRX.CH_MIN;
CH_MAX = RCRX.CH_MAX;
CH_TRIM = RCRX.CH_TRIM;
CH_DZ = RCRX.CH_DZ;
CH_REV = RCRX.CH_REV;
%--------------------------------------------------------------
% SCALING PARAMETERS
% Open-loop RC scale {'COM MOTOR VOLT','DIFF MOTOR VOLT'}
OPL_RC_SCALE = CONTROL.PARAM.OPL_RC_SCALE;
% Velocity RC scale {'FORWARD VEL REF','YAW RATE REF'}
VEL_RC_SCALE = CONTROL.PARAM.VEL_RC_SCALE;
% Wall follower RC scale {'FORWARD VEL REF','WALL DIST REF'}
WFL_RC_SCALE = CONTROL.PARAM.WFL_RC_SCALE;
%--------------------------------------------------------------
% CHANNEL SCALING
% RC_CH_TRIM saturation
CH_TRIM = CH_TRIM.*(CH_TRIM>=CH_MIN & CH_TRIM<=CH_MAX) ...
           + CH_MIN.*(CH_TRIM<CH_MIN) + CH_MAX.*(CH_TRIM>CH_MAX);
% Slope computation       
INC_UP = CH_MAX - CH_TRIM;
INC_DOWN = CH_TRIM - CH_MIN;
SLOPE = (INC_UP >= INC_DOWN).*(1+INC_DOWN./INC_UP)./(CH_MAX-CH_MIN) + ...
        (INC_UP < INC_DOWN).*(1+INC_UP./(INC_DOWN+sqrt(eps)))./(CH_MAX-CH_MIN);
% Dead zone
INC_CH_RAW = double(CH_RAW) - CH_TRIM;
INC_CH_RAW = INC_CH_RAW.*(abs(INC_CH_RAW)>CH_DZ);
% Scaled channels
CH_SCALED = 1e4*CH_REV.*SLOPE.*INC_CH_RAW;
% Change to pu 
CH_PU = 1e-4*CH_SCALED;
CH_PU = CH_PU.*(CH_PU>=-1 & CH_PU<=1) + (CH_PU>1);          
% Throttle channel between 0 and 1                        
CH_PU(4) = CH_PU(4)*(CH_PU(4)>=0 && CH_PU(4)<=1) + (CH_PU(4)>1);   
%--------------------------------------------------------------
% TARGET DEFINITION
switch CONTROL.STATE.CONTROL_MODE 
    case 0 % OPEN LOOP
        % {'MOTOR VOLT LEFT','MOTOR VOLT RIGHT'}
        if CONTROL.STATE.OPL_TARGET_SOURCE(1)==1 % JOYSTICK
            CONTROL.TARGET.OPL_REF_RC(1) = CH_PU(3)*OPL_RC_SCALE(1);
        end
        if CONTROL.STATE.OPL_TARGET_SOURCE(2)==1 % JOYSTICK
            CONTROL.TARGET.OPL_REF_RC(2) = CH_PU(2)*OPL_RC_SCALE(1);
        end
        if CONTROL.STATE.OPL_TARGET_SOURCE(1)==2 % SWITCH
            CONTROL.TARGET.OPL_REF_RC(1) = CONTROL.PARAM.OPL_RC_SWITCH(1,uint8(1+CH_PU(5)));
        end
        if CONTROL.STATE.OPL_TARGET_SOURCE(2)==2 % SWITCH
            CONTROL.TARGET.OPL_REF_RC(2) = CONTROL.PARAM.OPL_RC_SWITCH(2,uint8(1+CH_PU(6)));
        end       
    case 1 % VELOCITY CONTROL
        % {'FORWARD VEL REF','YAW RATE REF'}
        if CONTROL.STATE.VEL_TARGET_SOURCE(1)==1 % JOYSTICK
            CONTROL.TARGET.VEL_REF_RC(1) = CH_PU(3)*VEL_RC_SCALE(1);
        end
        if CONTROL.STATE.VEL_TARGET_SOURCE(2)==1 % JOYSTICK
            CONTROL.TARGET.VEL_REF_RC(2) = CH_PU(2)*VEL_RC_SCALE(1);
        end
        if CONTROL.STATE.VEL_TARGET_SOURCE(1)==2 % SWITCH
            CONTROL.TARGET.VEL_REF_RC(1) = CONTROL.PARAM.VEL_RC_SWITCH(1,uint8(1+CH_PU(5)));
        end
        if CONTROL.STATE.ATT_TARGET_SOURCE(2)==2 % SWITCH
            CONTROL.TARGET.VEL_REF_RC(2) = CONTROL.PARAM.VEL_RC_SWITCH(2,uint8(1+CH_PU(6)));
        end
    case 2 % WALL FOLLOWER
        % {'FORWARD VEL REF','WALL DIST REF'}
        if CONTROL.STATE.WFL_TARGET_SOURCE(1)==1 % JOYSTICK
            CONTROL.TARGET.WFL_REF_RC(1) = CH_PU(4)*WFL_RC_SCALE(1);
        end
        if CONTROL.STATE.WFL_TARGET_SOURCE(2)==1 % JOYSTICK
            CONTROL.TARGET.WFL_REF_RC(2) = CH_PU(2)*WFL_RC_SCALE(1);
        end
        if CONTROL.STATE.WFL_TARGET_SOURCE(1)==2 % SWITCH
            CONTROL.TARGET.WFL_REF_RC(1) = CONTROL.PARAM.WFL_RC_SWITCH(1,uint8(1+CH_PU(5)));
        end
        if CONTROL.STATE.WFL_TARGET_SOURCE(2)==2 % SWITCH
            CONTROL.TARGET.WFL_REF_RC(2) = CONTROL.PARAM.WFL_RC_SWITCH(2,uint8(1+CH_PU(6)));
        end
end
%--------------------------------------------------------------
% CONTROL BUS UPDATE
% RC CHANNELS (pu): channel range [-1 1] / Throtle range (channel 4) [0 1] 
CONTROL.TARGET.RC_CHANNELS = CH_PU(:);

== matlab function TEST_LIDAR/HARDWARE/COMMUNICATIONS/UART_MUX/RCRX iBUS/MATLAB Function ==
  data: iBUS_DATA input; CH_RAW output size=14
function CH_RAW = iBUS_DECODER(iBUS_DATA)
%--------------------------------------------------------------
persistent initialize CH_RAW_PREV
if isempty(initialize)
    initialize = 1;
    CH_RAW_PREV = uint16(1500*ones(14,1));
end
%--------------------------------------------------------------
% iBUS protocol: 14 channels uint16 in the range [1000 - 2000]
%--------------------------------------------------------------
% HEADER DETECTION
header = uint8([32 64]);
AUX1 = (iBUS_DATA == header(1));
AUX2 = (iBUS_DATA == header(2));
AUX3 = AUX1(1:end-1) & AUX2(2:end);
[max_value,index] = max(AUX3);
%--------------------------------------------------------------
% CHANNEL DETECTION
if max_value && ((index(1)+2+2*14-1)<=length(iBUS_DATA))
    CH_DATA = iBUS_DATA((index(1)+2):(index(1)+2+2*14-1));
    CH_LSB = uint16(CH_DATA(1:2:length(CH_DATA)));
    CH_MSB = uint16(CH_DATA(2:2:length(CH_DATA)));
    CH_RAW_AUX = uint16(CH_MSB*2^8 + CH_LSB);
    CH_RAW_PREV = CH_RAW_AUX;
else
    CH_RAW_AUX = CH_RAW_PREV;
end
%--------------------------------------------------------------
% CHANNELS 3 AND 4 ARE INTERCHANGED
CH_RAW = CH_RAW_AUX;
CH_RAW(3) = CH_RAW_AUX(4);
CH_RAW(4) = CH_RAW_AUX(3);
%--------------------------------------------------------------

return

== matlab function TEST_LIDAR/CONTROL/LOCAL TARGETS/FORWARD VELOCITY TARGET/RAMP ==
  data: SAMPLING_TIME input; ramp_out output
function ramp_out = RAMP(SAMPLING_TIME)

%--------------------------------------------------------------
% PERSISTENT VARIABLES
%--------------------------------------------------------------
persistent ramp ramp_slope TIMER initialize
if isempty(initialize)
    TIMER = 0;
    ramp = 1;
    ramp_slope = -1;
    initialize = 1;
end

TIMER = TIMER + SAMPLING_TIME;
if TIMER < 30
    ramp_out = ramp; 
    return
else
    TIMER = 0;
end

if ramp==1 || ramp==4
    ramp_slope = -ramp_slope;
end

ramp = ramp + ramp_slope;

ramp_out = ramp;

== matlab function TEST_LIDAR/HARDWARE/SENSORS/CURRENT_ADC_MCP3201_SPI/ADC UPDATE ==
  data: CONTROL_IN input Bus: CONTROL_Bus; VREF input; CONTROL output Bus: CONTROL_Bus; NBITS input; R_SHUNT input; ADC_CODE input
function CONTROL = ADC_UPDATE(CONTROL_IN,VREF,NBITS,R_SHUNT,ADC_CODE)

%% ACTUATOR BUS UPDATE
CONTROL = CONTROL_IN;

%% ADC CODE
AUX = dec2bin(ADC_CODE,16);
ADC_CODE = bin2dec(AUX(4:4+11));
ADC_VOLTAGE = VREF/2^NBITS*double(ADC_CODE);
ADC_CURRENT = ADC_VOLTAGE/R_SHUNT;
CONTROL.INPUT.CHARGING_CURRENT = ADC_CURRENT;

== matlab function TEST_LIDAR/SIMULATION/READ IMU/GRAVITY ROTATION ==
  data: PITCH_OFFSET input; GRAVITY_VECTOR output; GRAVITY input; VEHICLE_MODE input
function GRAVITY_VECTOR = GRAVITY_ROTATION(PITCH_OFFSET,GRAVITY,VEHICLE_MODE)
if VEHICLE_MODE
    ROTATION_MATRIX = [cos(PITCH_OFFSET) 0 -sin(PITCH_OFFSET) ; 0 1 0 ; sin(PITCH_OFFSET) 0 cos(PITCH_OFFSET)];
    GRAVITY_VECTOR = ROTATION_MATRIX*[GRAVITY ; 0 ; 0];
else
    GRAVITY_VECTOR = [0 ; 0 ; -GRAVITY];
end

== matlab function TEST_LIDAR/HARDWARE/ACTUATORS/MD25_I2C/READ MOTOR ENCODER/READ_ENCODER OLD ==
  data: CONTROL_IN input Bus: CONTROL_Bus; MOTOR_ENC_BYTES input; CONTROL output Bus: CONTROL_Bus
function CONTROL = READ_ENCODER(CONTROL_IN,MOTOR_ENC_BYTES)
%% UPDATE BUFFER
CONTROL = CONTROL_IN;

%--------------------------------------------------------------
% PARAMETERS
%--------------------------------------------------------------
% Sampling time (s)
SAMPLING_TIME = CONTROL.PARAM.SAMPLING_TIME;
% Encoder filter frequency (Hz)
ENC_FILT_FREQ = CONTROL.PARAM.ENC_FILT_FREQ;
% Distance between wheeels (m)
WHEEL_DIST = CONTROL.PARAM.WHEEL_DISTANCE;
% Wheel radius (m)
WHEEL_RADIUS = CONTROL.PARAM.WHEEL_RADIUS;
% Wheel gear ratio
WHEEL_GEAR_RATIO = CONTROL.PARAM.WHEEL_GEAR_RATIO;
% Motor gear ratio
MOTOR_GEAR_RATIO = CONTROL.PARAM.MOTOR_GEAR_RATIO;
% Encoder resolution: number of pulses / revolution of main shaft
MOTOR_ENC_RES = CONTROL.PARAM.MOTOR_ENC_RES; 

%--------------------------------------------------------------
% ENCODER READOUT
%--------------------------------------------------------------
right_enc = -double(typecast(MOTOR_ENC_BYTES([4 3 2 1],1),'int32'));
left_enc = -double(typecast(MOTOR_ENC_BYTES([8 7 6 5],1),'int32'));

%--------------------------------------------------------------
% STATE
%--------------------------------------------------------------
persistent initialize ENC_PREV INC_ENC_FILT YAW_ANGLE YAW_ANGLE_FILT...
           YAW_RATE YAW_RATE_FILT
N = 15;
if isempty(initialize)
    ENC_PREV = zeros(2,N); % N previous encoder measurements
    INC_ENC_FILT = zeros(2,1); % Filtered incremental encoder
    YAW_ANGLE = 0;
    YAW_RATE = 0;
    YAW_ANGLE_FILT = 0;
    YAW_RATE_FILT = 0;
    initialize = 1;
end

%--------------------------------------------------------------
% ENCODER FILTERING
%--------------------------------------------------------------
% Define incremental encoder threshold (deg)
THR_INC_ENC_DEG = 2/WHEEL_RADIUS*180/pi*SAMPLING_TIME; % 23 deg
% LPF discrete-time pole
ALFA = exp(-SAMPLING_TIME*2*pi*ENC_FILT_FREQ);
% Current encoder measurements (deg)
ENC_K = 360/MOTOR_ENC_RES/MOTOR_GEAR_RATIO/WHEEL_GEAR_RATIO*[left_enc ; right_enc];
% FIRST-ORDER INCREMENTAL SIGNALS (deg)
INC_ENC_NOW = [ENC_K ENC_PREV(:,1:end-1)]-ENC_PREV; % N samples
% OUTLIERS ARE ELIMINATED IN FIRST-ORDER INCREMENTAL SIGNALS
INC_ENC_MOD = INC_ENC_NOW; 
for nn=N-1:-1:1
  INC_ENC_MOD(:,nn) = INC_ENC_NOW(:,nn).*(abs(INC_ENC_NOW(:,nn))<=THR_INC_ENC_DEG) + INC_ENC_MOD(:,nn+1).*(abs(INC_ENC_NOW(:,nn))>THR_INC_ENC_DEG);
end
INC_ENC_MOD = INC_ENC_MOD(:,1:N-1); % N-1 samples
% UPDATE ENCODER MEMORY
ENC_PREV = [ENC_K ENC_PREV(:,1:end-1)];2
% FINAL INCREMENTAL ENCODER
INC_ENC = zeros(2,1);
INC_ENC(1) = INC_ENC_MOD(1,1);
INC_ENC(2) = INC_ENC_MOD(2,1);
% ALFA_FILTER
INC_ENC_FILT = ALFA*INC_ENC_FILT + (1-ALFA)*INC_ENC;  

%--------------------------------------------------------------
% FORWARD VEL
%--------------------------------------------------------------
FORWARD_VEL = mean(INC_ENC)/SAMPLING_TIME*pi/180*WHEEL_RADIUS;
FORWARD_VEL_FILT = mean(INC_ENC_FILT)/SAMPLING_TIME*pi/180*WHEEL_RADIUS;

%--------------------------------------------------------------
% YAW RATE
%--------------------------------------------------------------
YAW_RATE_PRV = YAW_RATE;
YAW_RATE_PRV_FILT = YAW_RATE_FILT;
YAW_RATE = (INC_ENC(1)-INC_ENC(2))/SAMPLING_TIME*pi/180*WHEEL_RADIUS/WHEEL_DIST;
YAW_RATE_FILT = (INC_ENC_FILT(1)-INC_ENC_FILT(2))/SAMPLING_TIME*pi/180*WHEEL_RADIUS/WHEEL_DIST;

%--------------------------------------------------------------
% YAW ANGLE
%--------------------------------------------------------------
YAW_ANGLE_PRV = YAW_ANGLE;
YAW_ANGLE_PRV_FILT = YAW_ANGLE_FILT;
YAW_ANGLE = YAW_ANGLE_PRV + SAMPLING_TIME/2*(YAW_RATE + YAW_RATE_PRV);
YAW_ANGLE_FILT = YAW_ANGLE_PRV_FILT + SAMPLING_TIME/2*(YAW_RATE_FILT + YAW_RATE_PRV_FILT);

%--------------------------------------------------------------
% MOTOR RATE
%--------------------------------------------------------------
MOTOR_RATE = INC_ENC/SAMPLING_TIME*pi/180*WHEEL_GEAR_RATIO;
MOTOR_RATE_FILT = INC_ENC_FILT/SAMPLING_TIME*pi/180*WHEEL_GEAR_RATIO;
MOTOR_RATE_CD = [sum(MOTOR_RATE) -diff(MOTOR_RATE)]/2*WHEEL_GEAR_RATIO;
MOTOR_RATE_CD_FILT = [sum(MOTOR_RATE_FILT) -diff(MOTOR_RATE_FILT)]/2*WHEEL_GEAR_RATIO;

%--------------------------------------------------------------
% UPDATE CONTROL BUS
%--------------------------------------------------------------
CONTROL.INPUT.ENC_FORWARD_VEL = FORWARD_VEL;
CONTROL.INPUT.ENC_FORWARD_VEL_FILT = FORWARD_VEL_FILT;
CONTROL.INPUT.ENC_YAW_RATE = YAW_RATE;
CONTROL.INPUT.ENC_YAW_RATE_FILT = YAW_RATE_FILT;
CONTROL.INPUT.ENC_YAW_ANG = YAW_ANGLE;
CONTROL.INPUT.ENC_YAW_ANG_FILT = YAW_ANGLE_FILT;
CONTROL.INPUT.ENC_MOTOR_RATE = MOTOR_RATE;
CONTROL.INPUT.ENC_MOTOR_RATE_FILT = MOTOR_RATE_FILT;
CONTROL.INPUT.ENC_MOTOR_RATE_CD = MOTOR_RATE_CD';
CONTROL.INPUT.ENC_MOTOR_RATE_CD_FILT = MOTOR_RATE_CD_FILT';
CONTROL.INPUT.ENC_MOTOR_ANG = pi/180*ENC_K;

return
